simulink model "ode"  (R2019b)
settings: Solver=FixedStepAuto  StartTime=0.0  StopTime=100  FixedStep=.01  RelTol=1e-3
settings Model: Creator=Rashedul Islam  LastModifiedBy=Rashedul Islam

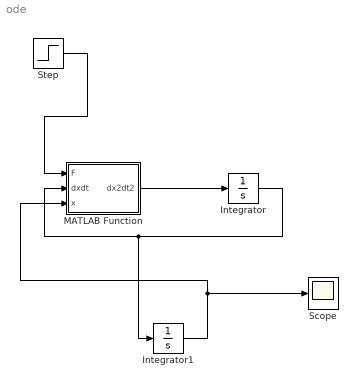
== system ode ==
  Integrator : Integrator
  Integrator1 : Integrator
  MATLAB Function : MATLAB Function  TreatAsAtomicUnit=on
  Scope : Scope
  Step : Step  SampleTime=0
  wires:
  MATLAB Function/1(dx2dt2) -> Integrator/1
  Integrator/1 -> Integrator1/1, MATLAB Function/2(dxdt)
  Integrator1/1 -> Scope/1, MATLAB Function/3(x)
  Step/1 -> MATLAB Function/1(F)

== matlab function ode/MATLAB Function ==
  data: F input; dx2dt2 output; dxdt input; x input
function dx2dt2 = fcn(F,dxdt,x)
M=1;
b=1;
k=20;
dx2dt2 = (F-b*dxdt-k*x)/M;
